simulink model "model"  (R2022b)
settings: Solver=VariableStepAuto  StartTime=0.0  StopTime=15  RelTol=1e-3
libraries: neural x114, simulink x4
(part 2 of 4)

== system model/level=2，训练时间15s，隐藏层15/Layer 1/Delays 1 ==
  "p{1}" : Inport  PortDimensions=8
      mask Display: e = 0.06;c1 = [120 230 180]/255;c2 = ([120 230 180]+0)/(256+128);c3 = ([120 230 180]+128)/(256+128);patch([0 1 1 0],[0 0 1 1],c1);patch([0 1 1 1-e 1-e 0+e],[0 0 1 1-e 0+e 0+e],c2);patch([0 0 1 1-e 0+e 0+e],[0 1 1 1-e 1-e 0+e],c3);plot([0 1 1 0 0],[0 0 1 1 0]);
  mux : Mux  Inputs=1
      mask Display: e = 0.06;c1 = [120 150 230]/255;c2 = ([120 150 230]+0)/383;c3 = ([120 150 230]+128)/383;patch([0 1 1 0],[0 0 1 1],c1);patch([0 1 1 1-e 1-e 0+e],[0 0 1 1-e 0+e 0+e],c2);patch([0 0 1 1-e 0+e 0+e],[0 1 1 1-e 1-e 0+e],c3);plot([0 1 1 0 0],[0 0 1 1 0]);disp('Mux')
  "pd{1,1}" : Outport
      mask Display: e = 0.06;c1 = [120 230 180]/255;c2 = ([120 230 180]+0)/(256+128);c3 = ([120 230 180]+128)/(256+128);patch([0 1 1 0],[0 0 1 1],c1);patch([0 1 1 1-e 1-e 0+e],[0 0 1 1-e 0+e 0+e],c2);patch([0 0 1 1-e 0+e 0+e],[0 1 1 1-e 1-e 0+e],c3);plot([0 1 1 0 0],[0 0 1 1 0]);
  wires:
  "p{1}"/1 -> mux/1
  mux/1 -> "pd{1,1}"/1

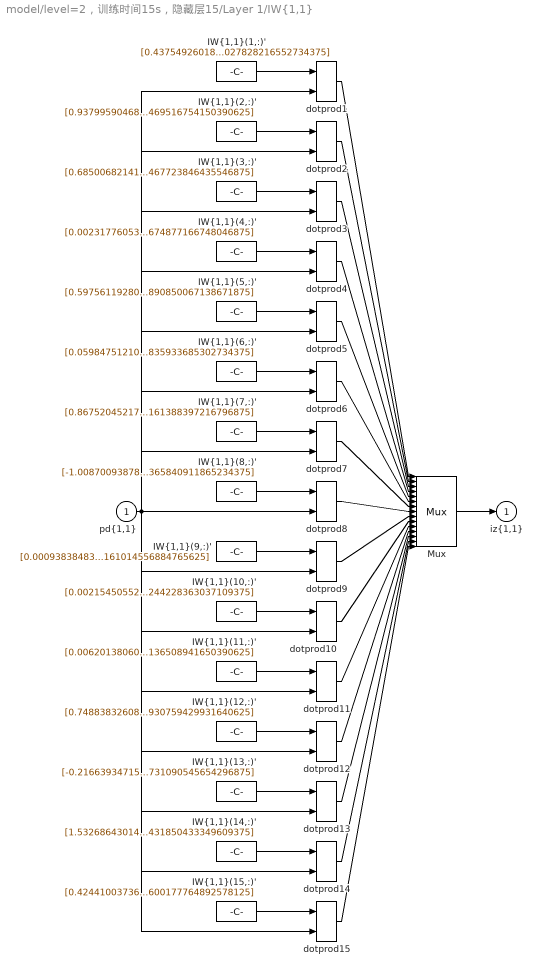
== system model/level=2，训练时间15s，隐藏层15/Layer 1/IW{1,1} ==
  "pd{1,1}" : Inport  PortDimensions=8
      mask Display: e = 0.06;c1 = [120 230 180]/255;c2 = ([120 230 180]+0)/(256+128);c3 = ([120 230 180]+128)/(256+128);patch([0 1 1 0],[0 0 1 1],c1);patch([0 1 1 1-e 1-e 0+e],[0 0 1 1-e 0+e 0+e],c2);patch([0 0 1 1-e 0+e 0+e],[0 1 1 1-e 1-e 0+e],c3);plot([0 1 1 0 0],[0 0 1 1 0]);
  "IW{1,1}(1,:)'" : Constant  Value=[0.437549260188033473095714498413144610822200775146484375;-0.543752134402809783608745419769547879695892333984375;-0.77263238466385486535870086299837566912174224853515625;0.7440170273308268633627449162304401397705078125;-1.41516521745081202965366173884831368923187255859375;1.2537441253925447615102939380449242889881134033203125;0.904308850719730106249016898800618946552276611328125;-0.56373674454161937230622925198986195027828216552734375]
      mask Display: e = 0.06;c1 = [120 150 230]/255;c2 = ([120 150 230]+0)/383;c3 = ([120 150 230]+128)/383;patch([0 1 1 0],[0 0 1 1],c1);patch([0 1 1 1-e 1-e 0+e],[0 0 1 1-e 0+e 0+e],c2);patch([0 0 1 1-e 0+e 0+e],[0 1 1 1-e 1-e 0+e],c3);plot([0 1 1 0 0],[0 0 1 1 0]);disp('Weights');
  "IW{1,1}(10,:)'" : Constant  Value=[0.0021545055257757681106689506833617997472174465656280517578125;-0.000689327560344079183322907322661876605707220733165740966796875;0.0025722441794928919099605391096474704681895673274993896484375;0.01018820606628951554173401206071503111161291599273681640625;0.250021595562128828849068895578966476023197174072265625;0.405128587531441264335541063701384700834751129150390625;-0.09831810982660001141386629797125351615250110626220703125;-0.498693163090770885670366396880126558244228363037109375]
      mask Display: e = 0.06;c1 = [120 150 230]/255;c2 = ([120 150 230]+0)/383;c3 = ([120 150 230]+128)/383;patch([0 1 1 0],[0 0 1 1],c1);patch([0 1 1 1-e 1-e 0+e],[0 0 1 1-e 0+e 0+e],c2);patch([0 0 1 1-e 0+e 0+e],[0 1 1 1-e 1-e 0+e],c3);plot([0 1 1 0 0],[0 0 1 1 0]);disp('Weights');
  "IW{1,1}(11,:)'" : Constant  Value=[0.006201380606661944898394533964847141760401427745819091796875;0.0037383409814706852584975660391819474170915782451629638671875;0.0040645559789425182717348405958546209149062633514404296875;0.0276355472342307249833393001381409703753888607025146484375;0.10749327599186429826882971383383846841752529144287109375;1.5640527442188096873820768450968898832798004150390625;0.364238376530578611411925749052898027002811431884765625;-1.772260716698662807999653523438610136508941650390625]
      mask Display: e = 0.06;c1 = [120 150 230]/255;c2 = ([120 150 230]+0)/383;c3 = ([120 150 230]+128)/383;patch([0 1 1 0],[0 0 1 1],c1);patch([0 1 1 1-e 1-e 0+e],[0 0 1 1-e 0+e 0+e],c2);patch([0 0 1 1-e 0+e 0+e],[0 1 1 1-e 1-e 0+e],c3);plot([0 1 1 0 0],[0 0 1 1 0]);disp('Weights');
  "IW{1,1}(12,:)'" : Constant  Value=[0.7488383260876163571850838707177899777889251708984375;1.484571579328911372641641719383187592029571533203125;0.16446117310405139466666923908633179962635040283203125;0.1800313451031676781344259552497533150017261505126953125;1.4197521021375887340099097855272702872753143310546875;0.5167645863546084239459332820842973887920379638671875;-0.83653735985908939110089477253495715558528900146484375;-0.4654659156868492519976143739768303930759429931640625]
      mask Display: e = 0.06;c1 = [120 150 230]/255;c2 = ([120 150 230]+0)/383;c3 = ([120 150 230]+128)/383;patch([0 1 1 0],[0 0 1 1],c1);patch([0 1 1 1-e 1-e 0+e],[0 0 1 1-e 0+e 0+e],c2);patch([0 0 1 1-e 0+e 0+e],[0 1 1 1-e 1-e 0+e],c3);plot([0 1 1 0 0],[0 0 1 1 0]);disp('Weights');
  "IW{1,1}(13,:)'" : Constant  Value=[-0.2166393471563960171355489592315279878675937652587890625;-0.72288634706720411582381302650901488959789276123046875;0.76398367116674703591883144326857291162014007568359375;0.31702488552167162882966522374772466719150543212890625;1.61289116019904898990944275283254683017730712890625;-0.6538957185094822488480303945834748446941375732421875;-1.731230912011282985218940666527487337589263916015625;-1.03061719525024653165701238322071731090545654296875]
      mask Display: e = 0.06;c1 = [120 150 230]/255;c2 = ([120 150 230]+0)/383;c3 = ([120 150 230]+128)/383;patch([0 1 1 0],[0 0 1 1],c1);patch([0 1 1 1-e 1-e 0+e],[0 0 1 1-e 0+e 0+e],c2);patch([0 0 1 1-e 0+e 0+e],[0 1 1 1-e 1-e 0+e],c3);plot([0 1 1 0 0],[0 0 1 1 0]);disp('Weights');
  "IW{1,1}(14,:)'" : Constant  Value=[1.532686430143353373267700590076856315135955810546875;1.384326577376502331873098228243179619312286376953125;-0.66610376092964418415220961833256296813488006591796875;-0.68326384700084352719073876869515515863895416259765625;2.42772285085268624271748194587416946887969970703125;-1.7746665444950675549762308946810662746429443359375;-3.146294986981688079907826249836944043636322021484375;4.184593075317817323366398341022431850433349609375]
      mask Display: e = 0.06;c1 = [120 150 230]/255;c2 = ([120 150 230]+0)/383;c3 = ([120 150 230]+128)/383;patch([0 1 1 0],[0 0 1 1],c1);patch([0 1 1 1-e 1-e 0+e],[0 0 1 1-e 0+e 0+e],c2);patch([0 0 1 1-e 0+e 0+e],[0 1 1 1-e 1-e 0+e],c3);plot([0 1 1 0 0],[0 0 1 1 0]);disp('Weights');
  "IW{1,1}(15,:)'" : Constant  Value=[0.42441003736812199509387255602632649242877960205078125;-0.317624639112158824172382765027577988803386688232421875;0.6566292418801129571193087031133472919464111328125;0.354371501508666864044272415412706322968006134033203125;0.55838469564761428198806925138342194259166717529296875;0.634921241532747426816740698995999991893768310546875;0.855102081342001607566771781421266496181488037109375;-2.10814001639689241329733704333193600177764892578125]
      mask Display: e = 0.06;c1 = [120 150 230]/255;c2 = ([120 150 230]+0)/383;c3 = ([120 150 230]+128)/383;patch([0 1 1 0],[0 0 1 1],c1);patch([0 1 1 1-e 1-e 0+e],[0 0 1 1-e 0+e 0+e],c2);patch([0 0 1 1-e 0+e 0+e],[0 1 1 1-e 1-e 0+e],c3);plot([0 1 1 0 0],[0 0 1 1 0]);disp('Weights');
  "IW{1,1}(2,:)'" : Constant  Value=[0.93799590468169125045960754505358636379241943359375;0.0389757109661090506147473888631793670356273651123046875;1.225492864464332143370484118349850177764892578125;-1.40774598885113988444572896696627140045166015625;-0.54987653716072848464335720564122311770915985107421875;-2.160972880697380471559654324664734303951263427734375;-0.1067846054083453621874610917075187899172306060791015625;0.4523584479950049086482977145351469516754150390625]
      mask Display: e = 0.06;c1 = [120 150 230]/255;c2 = ([120 150 230]+0)/383;c3 = ([120 150 230]+128)/383;patch([0 1 1 0],[0 0 1 1],c1);patch([0 1 1 1-e 1-e 0+e],[0 0 1 1-e 0+e 0+e],c2);patch([0 0 1 1-e 0+e 0+e],[0 1 1 1-e 1-e 0+e],c3);plot([0 1 1 0 0],[0 0 1 1 0]);disp('Weights');
  "IW{1,1}(3,:)'" : Constant  Value=[0.685006821417439848431740756495855748653411865234375;-0.151121840928223838407262746841297484934329986572265625;-0.90905729353138209347662268555723130702972412109375;-0.9146870439134369146216840817942284047603607177734375;1.5466948145383672130748209383455105125904083251953125;-1.0684967037827195479593456184375099837779998779296875;-1.41530069117394763367201449000276625156402587890625;2.208804266633716206769122436526231467723846435546875]
      mask Display: e = 0.06;c1 = [120 150 230]/255;c2 = ([120 150 230]+0)/383;c3 = ([120 150 230]+128)/383;patch([0 1 1 0],[0 0 1 1],c1);patch([0 1 1 1-e 1-e 0+e],[0 0 1 1-e 0+e 0+e],c2);patch([0 0 1 1-e 0+e 0+e],[0 1 1 1-e 1-e 0+e],c3);plot([0 1 1 0 0],[0 0 1 1 0]);disp('Weights');
  "IW{1,1}(4,:)'" : Constant  Value=[0.00231776053848237011123512019139525364153087139129638671875;-0.000436669150460885385246767587119620657176710665225982666015625;0.0025125418369684950244125065665912188705988228321075439453125;0.01191060627903158843088338159077466116286814212799072265625;0.53703993975591324261387171645765192806720733642578125;1.4164231725934055550197854245197959244251251220703125;-0.237965122046671695432706883366336114704608917236328125;-1.035250733950956014695066187414340674877166748046875]
      mask Display: e = 0.06;c1 = [120 150 230]/255;c2 = ([120 150 230]+0)/383;c3 = ([120 150 230]+128)/383;patch([0 1 1 0],[0 0 1 1],c1);patch([0 1 1 1-e 1-e 0+e],[0 0 1 1-e 0+e 0+e],c2);patch([0 0 1 1-e 0+e 0+e],[0 1 1 1-e 1-e 0+e],c3);plot([0 1 1 0 0],[0 0 1 1 0]);disp('Weights');
  "IW{1,1}(5,:)'" : Constant  Value=[0.59756119280919561820297758458764292299747467041015625;-0.6096022740572006881620836793445050716400146484375;-0.188502054741053637343384252744726836681365966796875;-0.08490586213242155844138636666684760712087154388427734375;-0.227815400909060550294071845200960524380207061767578125;0.347143384643888663898536606211564503610134124755859375;-1.9577073019096020711771188871352933347225189208984375;0.71978561343270797134863414612482301890850067138671875]
      mask Display: e = 0.06;c1 = [120 150 230]/255;c2 = ([120 150 230]+0)/383;c3 = ([120 150 230]+128)/383;patch([0 1 1 0],[0 0 1 1],c1);patch([0 1 1 1-e 1-e 0+e],[0 0 1 1-e 0+e 0+e],c2);patch([0 0 1 1-e 0+e 0+e],[0 1 1 1-e 1-e 0+e],c3);plot([0 1 1 0 0],[0 0 1 1 0]);disp('Weights');
  "IW{1,1}(6,:)'" : Constant  Value=[0.059847512100399909151793309547429089434444904327392578125;0.74983605040232192973093106047599576413631439208984375;-0.7210875241722394246579597165691666305065155029296875;1.047180192591222525066996240639127790927886962890625;0.07693879015290940037719025212936685420572757720947265625;1.741335040725929150795536770601756870746612548828125;0.07038197833113417345440865346972714178264141082763671875;0.09342308462036284788521101063452078960835933685302734375]
      mask Display: e = 0.06;c1 = [120 150 230]/255;c2 = ([120 150 230]+0)/383;c3 = ([120 150 230]+128)/383;patch([0 1 1 0],[0 0 1 1],c1);patch([0 1 1 1-e 1-e 0+e],[0 0 1 1-e 0+e 0+e],c2);patch([0 0 1 1-e 0+e 0+e],[0 1 1 1-e 1-e 0+e],c3);plot([0 1 1 0 0],[0 0 1 1 0]);disp('Weights');
  "IW{1,1}(7,:)'" : Constant  Value=[0.86752045217883433370076318169594742357730865478515625;-0.96548421997974731567637718399055302143096923828125;0.321899851156346006320063679595477879047393798828125;-1.0278579156471467914713002755888737738132476806640625;-0.1653280131719136736290209910293924622237682342529296875;1.3665634118383358508452829482848756015300750732421875;-0.653315092554610732378250759211368858814239501953125;-0.354784734114196698140375474395113997161388397216796875]
      mask Display: e = 0.06;c1 = [120 150 230]/255;c2 = ([120 150 230]+0)/383;c3 = ([120 150 230]+128)/383;patch([0 1 1 0],[0 0 1 1],c1);patch([0 1 1 1-e 1-e 0+e],[0 0 1 1-e 0+e 0+e],c2);patch([0 0 1 1-e 0+e 0+e],[0 1 1 1-e 1-e 0+e],c3);plot([0 1 1 0 0],[0 0 1 1 0]);disp('Weights');
  "IW{1,1}(8,:)'" : Constant  Value=[-1.0087009387896153089769768484984524548053741455078125;-0.89390992537081881419425144486012868583202362060546875;-1.1882265121192616685874554605106823146343231201171875;0.83809871162911953046403823464061133563518524169921875;-1.59123040137597282495107720023952424526214599609375;0.267739811475067812640560305226244963705539703369140625;2.231364372002818896589815267361700534820556640625;-0.58440227767868557773311977143748663365840911865234375]
      mask Display: e = 0.06;c1 = [120 150 230]/255;c2 = ([120 150 230]+0)/383;c3 = ([120 150 230]+128)/383;patch([0 1 1 0],[0 0 1 1],c1);patch([0 1 1 1-e 1-e 0+e],[0 0 1 1-e 0+e 0+e],c2);patch([0 0 1 1-e 0+e 0+e],[0 1 1 1-e 1-e 0+e],c3);plot([0 1 1 0 0],[0 0 1 1 0]);disp('Weights');
  "IW{1,1}(9,:)'" : Constant  Value=[0.000938384833547240893893148783178048688569106161594390869140625;-0.00012713226525252224632760167377654170195455662906169891357421875;0.000847236512902139614518415289268205015105195343494415283203125;0.005008163419334926529102869352527704904787242412567138671875;-0.65488636048362280916990130208432674407958984375;-0.158363103243627623140099558440851978957653045654296875;0.328358097555003503043025148144806735217571258544921875;-0.071767526744820619999387645293609239161014556884765625]
      mask Display: e = 0.06;c1 = [120 150 230]/255;c2 = ([120 150 230]+0)/383;c3 = ([120 150 230]+128)/383;patch([0 1 1 0],[0 0 1 1],c1);patch([0 1 1 1-e 1-e 0+e],[0 0 1 1-e 0+e 0+e],c2);patch([0 0 1 1-e 0+e 0+e],[0 1 1 1-e 1-e 0+e],c3);plot([0 1 1 0 0],[0 0 1 1 0]);disp('Weights');
  Mux : Mux  Inputs=15
      mask Display: e = 0.06;c1 = [120 150 230]/255;c2 = ([120 150 230]+0)/383;c3 = ([120 150 230]+128)/383;patch([0 1 1 0],[0 0 1 1],c1);patch([0 1 1 1-e 1-e 0+e],[0 0 1 1-e 0+e 0+e],c2);patch([0 0 1 1-e 0+e 0+e],[0 1 1 1-e 1-e 0+e],c3);plot([0 1 1 0 0],[0 0 1 1 0]);disp('Mux');
  dotprod{1..15} (15 alike) : neural/Weight Functions/dotprod
  "iz{1,1}" : Outport
      mask Display: e = 0.06;c1 = [120 230 180]/255;c2 = ([120 230 180]+0)/(256+128);c3 = ([120 230 180]+128)/(256+128);patch([0 1 1 0],[0 0 1 1],c1);patch([0 1 1 1-e 1-e 0+e],[0 0 1 1-e 0+e 0+e],c2);patch([0 0 1 1-e 0+e 0+e],[0 1 1 1-e 1-e 0+e],c3);plot([0 1 1 0 0],[0 0 1 1 0]);
  wires:
  "IW{1,1}(1,:)'"/1 -> dotprod1/1
  "pd{1,1}"/1 -> dotprod1/2, dotprod2/2, dotprod3/2, dotprod4/2, dotprod5/2, dotprod6/2, dotprod7/2, dotprod8/2, dotprod9/2, dotprod10/2, dotprod11/2, dotprod12/2, dotprod13/2, dotprod14/2, dotprod15/2
  dotprod1/1 -> Mux/1
  "IW{1,1}(2,:)'"/1 -> dotprod2/1
  dotprod2/1 -> Mux/2
  "IW{1,1}(3,:)'"/1 -> dotprod3/1
  dotprod3/1 -> Mux/3
  "IW{1,1}(4,:)'"/1 -> dotprod4/1
  dotprod4/1 -> Mux/4
  "IW{1,1}(5,:)'"/1 -> dotprod5/1
  dotprod5/1 -> Mux/5
  "IW{1,1}(6,:)'"/1 -> dotprod6/1
  dotprod6/1 -> Mux/6
  "IW{1,1}(7,:)'"/1 -> dotprod7/1
  dotprod7/1 -> Mux/7
  "IW{1,1}(8,:)'"/1 -> dotprod8/1
  dotprod8/1 -> Mux/8
  "IW{1,1}(9,:)'"/1 -> dotprod9/1
  dotprod9/1 -> Mux/9
  "IW{1,1}(10,:)'"/1 -> dotprod10/1
  dotprod10/1 -> Mux/10
  "IW{1,1}(11,:)'"/1 -> dotprod11/1
  dotprod11/1 -> Mux/11
  "IW{1,1}(12,:)'"/1 -> dotprod12/1
  dotprod12/1 -> Mux/12
  "IW{1,1}(13,:)'"/1 -> dotprod13/1
  dotprod13/1 -> Mux/13
  "IW{1,1}(14,:)'"/1 -> dotprod14/1
  dotprod14/1 -> Mux/14
  "IW{1,1}(15,:)'"/1 -> dotprod15/1
  dotprod15/1 -> Mux/15
  Mux/1 -> "iz{1,1}"/1

== system model/level=2，训练时间15s，隐藏层15/Layer 2/Delays 1 ==
  "p{2}" : Inport  PortDimensions=15
      mask Display: e = 0.06;c1 = [120 230 180]/255;c2 = ([120 230 180]+0)/(256+128);c3 = ([120 230 180]+128)/(256+128);patch([0 1 1 0],[0 0 1 1],c1);patch([0 1 1 1-e 1-e 0+e],[0 0 1 1-e 0+e 0+e],c2);patch([0 0 1 1-e 0+e 0+e],[0 1 1 1-e 1-e 0+e],c3);plot([0 1 1 0 0],[0 0 1 1 0]);
  mux : Mux  Inputs=1
      mask Display: e = 0.06;c1 = [120 150 230]/255;c2 = ([120 150 230]+0)/383;c3 = ([120 150 230]+128)/383;patch([0 1 1 0],[0 0 1 1],c1);patch([0 1 1 1-e 1-e 0+e],[0 0 1 1-e 0+e 0+e],c2);patch([0 0 1 1-e 0+e 0+e],[0 1 1 1-e 1-e 0+e],c3);plot([0 1 1 0 0],[0 0 1 1 0]);disp('Mux')
  "pd{2,1}" : Outport
      mask Display: e = 0.06;c1 = [120 230 180]/255;c2 = ([120 230 180]+0)/(256+128);c3 = ([120 230 180]+128)/(256+128);patch([0 1 1 0],[0 0 1 1],c1);patch([0 1 1 1-e 1-e 0+e],[0 0 1 1-e 0+e 0+e],c2);patch([0 0 1 1-e 0+e 0+e],[0 1 1 1-e 1-e 0+e],c3);plot([0 1 1 0 0],[0 0 1 1 0]);
  wires:
  "p{2}"/1 -> mux/1
  mux/1 -> "pd{2,1}"/1

== system model/level=2，训练时间15s，隐藏层15/Layer 2/LW{2,1} ==
  "ad{2,1}" : Inport  PortDimensions=15
      mask Display: e = 0.06;c1 = [120 230 180]/255;c2 = ([120 230 180]+0)/(256+128);c3 = ([120 230 180]+128)/(256+128);patch([0 1 1 0],[0 0 1 1],c1);patch([0 1 1 1-e 1-e 0+e],[0 0 1 1-e 0+e 0+e],c2);patch([0 0 1 1-e 0+e 0+e],[0 1 1 1-e 1-e 0+e],c3);plot([0 1 1 0 0],[0 0 1 1 0]);
  "IW{2,1}(1,:)'" : Constant  Value=[0.000348521019966015134679271358919550038990564644336700439453125;-0.00105511526222962464909016500058669407735578715801239013671875;-0.0004875548366492649652627344725175362327718175947666168212890625;-1.1162096356705231148254142681253142654895782470703125;0.000566277605183764984851657597886287476285360753536224365234375;0.000434593678046664758617134705076523459865711629390716552734375;-0.0003371799056245722465974257175957973231561481952667236328125;0.00021859886636651514632383175307239753237809054553508758544921875;-2.87625249739135568916026386432349681854248046875;2.514252278515631378041916832444258034229278564453125;0.346485318185967783310985623757005669176578521728515625;0.000561811409637976810586834641725317851523868739604949951171875;0.00014173139297834577601635508425914622421259991824626922607421875;-0.00010903110141313854101509372984679657747619785368442535400390625;-0.001096015330055519036711597635758153046481311321258544921875]
      mask Display: e = 0.06;c1 = [120 150 230]/255;c2 = ([120 150 230]+0)/383;c3 = ([120 150 230]+128)/383;patch([0 1 1 0],[0 0 1 1],c1);patch([0 1 1 1-e 1-e 0+e],[0 0 1 1-e 0+e 0+e],c2);patch([0 0 1 1-e 0+e 0+e],[0 1 1 1-e 1-e 0+e],c3);plot([0 1 1 0 0],[0 0 1 1 0]);disp('weights');
  "IW{2,1}(2,:)'" : Constant  Value=[-0.000118459432783138453857720018280730300830327905714511871337890625;0.00109455608219046775751726041647771126008592545986175537109375;0.000248773173976225663028838397394792991690337657928466796875;2.376139494105127258904985865228809416294097900390625;-0.00060637236490409629312281492019565121154300868511199951171875;-0.000489683042123572405575349097972548406687565147876739501953125;0.00023224171170072960106167681004762926022522151470184326171875;-0.0002224587961179582090535944427500680831144563853740692138671875;0.76265316778717873180681863232166506350040435791015625;-2.917666926702186191988630525884218513965606689453125;-0.389603751198402570299350600180332548916339874267578125;-0.000526230007708676397575053851340953769977204501628875732421875;-0.000272639471284036728586375186722534635919146239757537841796875;0.0001435751291894367159991674487429236251045949757099151611328125;0.001218926641691715773152537849455256946384906768798828125]
      mask Display: e = 0.06;c1 = [120 150 230]/255;c2 = ([120 150 230]+0)/383;c3 = ([120 150 230]+128)/383;patch([0 1 1 0],[0 0 1 1],c1);patch([0 1 1 1-e 1-e 0+e],[0 0 1 1-e 0+e 0+e],c2);patch([0 0 1 1-e 0+e 0+e],[0 1 1 1-e 1-e 0+e],c3);plot([0 1 1 0 0],[0 0 1 1 0]);disp('weights');
  Mux : Mux  Inputs=2
      mask Display: e = 0.06;c1 = [120 150 230]/255;c2 = ([120 150 230]+0)/383;c3 = ([120 150 230]+128)/383;patch([0 1 1 0],[0 0 1 1],c1);patch([0 1 1 1-e 1-e 0+e],[0 0 1 1-e 0+e 0+e],c2);patch([0 0 1 1-e 0+e 0+e],[0 1 1 1-e 1-e 0+e],c3);plot([0 1 1 0 0],[0 0 1 1 0]);disp('Mux');
  dotprod1 : neural/Weight Functions/dotprod
  dotprod2 : neural/Weight Functions/dotprod
  "lz{2,1}" : Outport
      mask Display: e = 0.06;c1 = [120 230 180]/255;c2 = ([120 230 180]+0)/(256+128);c3 = ([120 230 180]+128)/(256+128);patch([0 1 1 0],[0 0 1 1],c1);patch([0 1 1 1-e 1-e 0+e],[0 0 1 1-e 0+e 0+e],c2);patch([0 0 1 1-e 0+e 0+e],[0 1 1 1-e 1-e 0+e],c3);plot([0 1 1 0 0],[0 0 1 1 0]);
  wires:
  "IW{2,1}(1,:)'"/1 -> dotprod1/1
  "ad{2,1}"/1 -> dotprod1/2, dotprod2/2
  dotprod1/1 -> Mux/1
  "IW{2,1}(2,:)'"/1 -> dotprod2/1
  dotprod2/1 -> Mux/2
  Mux/1 -> "lz{2,1}"/1

== system model/level=2，训练时间15s，隐藏层30/Layer 1/Delays 1 ==
  "p{1}" : Inport  PortDimensions=8
      mask Display: e = 0.06;c1 = [120 230 180]/255;c2 = ([120 230 180]+0)/(256+128);c3 = ([120 230 180]+128)/(256+128);patch([0 1 1 0],[0 0 1 1],c1);patch([0 1 1 1-e 1-e 0+e],[0 0 1 1-e 0+e 0+e],c2);patch([0 0 1 1-e 0+e 0+e],[0 1 1 1-e 1-e 0+e],c3);plot([0 1 1 0 0],[0 0 1 1 0]);
  mux : Mux  Inputs=1
      mask Display: e = 0.06;c1 = [120 150 230]/255;c2 = ([120 150 230]+0)/383;c3 = ([120 150 230]+128)/383;patch([0 1 1 0],[0 0 1 1],c1);patch([0 1 1 1-e 1-e 0+e],[0 0 1 1-e 0+e 0+e],c2);patch([0 0 1 1-e 0+e 0+e],[0 1 1 1-e 1-e 0+e],c3);plot([0 1 1 0 0],[0 0 1 1 0]);disp('Mux')
  "pd{1,1}" : Outport
      mask Display: e = 0.06;c1 = [120 230 180]/255;c2 = ([120 230 180]+0)/(256+128);c3 = ([120 230 180]+128)/(256+128);patch([0 1 1 0],[0 0 1 1],c1);patch([0 1 1 1-e 1-e 0+e],[0 0 1 1-e 0+e 0+e],c2);patch([0 0 1 1-e 0+e 0+e],[0 1 1 1-e 1-e 0+e],c3);plot([0 1 1 0 0],[0 0 1 1 0]);
  wires:
  "p{1}"/1 -> mux/1
  mux/1 -> "pd{1,1}"/1

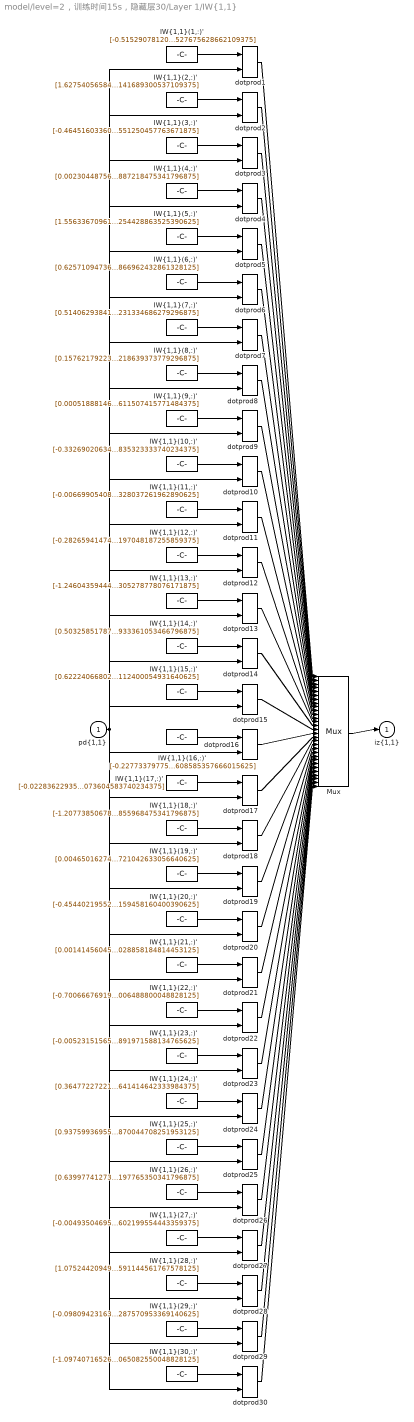
== system model/level=2，训练时间15s，隐藏层30/Layer 1/IW{1,1} ==
  "pd{1,1}" : Inport  PortDimensions=8
      mask Display: e = 0.06;c1 = [120 230 180]/255;c2 = ([120 230 180]+0)/(256+128);c3 = ([120 230 180]+128)/(256+128);patch([0 1 1 0],[0 0 1 1],c1);patch([0 1 1 1-e 1-e 0+e],[0 0 1 1-e 0+e 0+e],c2);patch([0 0 1 1-e 0+e 0+e],[0 1 1 1-e 1-e 0+e],c3);plot([0 1 1 0 0],[0 0 1 1 0]);
  "IW{1,1}(1,:)'" : Constant  Value=[-0.51529078120398874585106341328355483710765838623046875;-0.358908036286977927264985055444412864744663238525390625;-0.6444010451648869430840704808360897004604339599609375;1.0071702189204874144934365176595747470855712890625;0.02248108230128505191647292349443887360394001007080078125;0.26389261957038900874294995446689426898956298828125;-1.39021552883888066531881122500635683536529541015625;1.2659727968487819449450171305215917527675628662109375]
      mask Display: e = 0.06;c1 = [120 150 230]/255;c2 = ([120 150 230]+0)/383;c3 = ([120 150 230]+128)/383;patch([0 1 1 0],[0 0 1 1],c1);patch([0 1 1 1-e 1-e 0+e],[0 0 1 1-e 0+e 0+e],c2);patch([0 0 1 1-e 0+e 0+e],[0 1 1 1-e 1-e 0+e],c3);plot([0 1 1 0 0],[0 0 1 1 0]);disp('Weights');
  "IW{1,1}(10,:)'" : Constant  Value=[-0.332690206349311623501563417448778636753559112548828125;-0.446190121055760169355153266224078834056854248046875;-0.66273204507507565974577801171108148992061614990234375;0.28187276867938881874664502902305684983730316162109375;-0.189171155935518309210152665400528348982334136962890625;1.6197350687076081943160943410475738346576690673828125;0.56871889947271869747424943852820433676242828369140625;-0.255758907890911879601247846949263475835323333740234375]
      mask Display: e = 0.06;c1 = [120 150 230]/255;c2 = ([120 150 230]+0)/383;c3 = ([120 150 230]+128)/383;patch([0 1 1 0],[0 0 1 1],c1);patch([0 1 1 1-e 1-e 0+e],[0 0 1 1-e 0+e 0+e],c2);patch([0 0 1 1-e 0+e 0+e],[0 1 1 1-e 1-e 0+e],c3);plot([0 1 1 0 0],[0 0 1 1 0]);disp('Weights');
  "IW{1,1}(11,:)'" : Constant  Value=[-0.00669905408885207616365153882043159683234989643096923828125;7.324578259464768997637207359474587065051309764385223388671875e-05;0.005122104765875284786147414450852011214010417461395263671875;0.0044576255094989185312481794198902207426726818084716796875;-0.61000919335633485562908617794164456427097320556640625;0.87083644538918825173112736592884175479412078857421875;1.41342271393398188905621282174251973628997802734375;0.2003239174094197105890913235271000303328037261962890625]
      mask Display: e = 0.06;c1 = [120 150 230]/255;c2 = ([120 150 230]+0)/383;c3 = ([120 150 230]+128)/383;patch([0 1 1 0],[0 0 1 1],c1);patch([0 1 1 1-e 1-e 0+e],[0 0 1 1-e 0+e 0+e],c2);patch([0 0 1 1-e 0+e 0+e],[0 1 1 1-e 1-e 0+e],c3);plot([0 1 1 0 0],[0 0 1 1 0]);disp('Weights');
  "IW{1,1}(12,:)'" : Constant  Value=[-0.282659414743081705001515047115390188992023468017578125;-0.0262903330688668800119156543360077193938195705413818359375;-0.1239076488234570894153563358486280776560306549072265625;1.21520544753379855507091633626259863376617431640625;0.703174536692124707570883401785977184772491455078125;0.640376888760982865278492681682109832763671875;0.42448921427386909765999689625459723174571990966796875;-0.02889564638400710094856549403630197048187255859375]
      mask Display: e = 0.06;c1 = [120 150 230]/255;c2 = ([120 150 230]+0)/383;c3 = ([120 150 230]+128)/383;patch([0 1 1 0],[0 0 1 1],c1);patch([0 1 1 1-e 1-e 0+e],[0 0 1 1-e 0+e 0+e],c2);patch([0 0 1 1-e 0+e 0+e],[0 1 1 1-e 1-e 0+e],c3);plot([0 1 1 0 0],[0 0 1 1 0]);disp('Weights');
  "IW{1,1}(13,:)'" : Constant  Value=[-1.246043594448879243685723849921487271785736083984375;0.79398157078300923839009328730753622949123382568359375;-1.02458216852873551516722727683372795581817626953125;-0.16469520201554488370021545051713474094867706298828125;0.81489123823356701681319691488170064985752105712890625;0.9886847587319078645151648743194527924060821533203125;-1.3453903888704521474295461302972398698329925537109375;0.53475340518652003662936067485134117305278778076171875]
      mask Display: e = 0.06;c1 = [120 150 230]/255;c2 = ([120 150 230]+0)/383;c3 = ([120 150 230]+128)/383;patch([0 1 1 0],[0 0 1 1],c1);patch([0 1 1 1-e 1-e 0+e],[0 0 1 1-e 0+e 0+e],c2);patch([0 0 1 1-e 0+e 0+e],[0 1 1 1-e 1-e 0+e],c3);plot([0 1 1 0 0],[0 0 1 1 0]);disp('Weights');
  "IW{1,1}(14,:)'" : Constant  Value=[0.50325851787219788580074464334757067263126373291015625;1.274005584053836681590610169223509728908538818359375;0.1542261287740250008670983561387402005493640899658203125;-0.66552405816708015695581934778601862490177154541015625;0.11153763735982609450747560231320676393806934356689453125;-1.22764307291851171299867928610183298587799072265625;1.20325230730118004629503047908656299114227294921875;0.60351869658145307351304609255748800933361053466796875]
      mask Display: e = 0.06;c1 = [120 150 230]/255;c2 = ([120 150 230]+0)/383;c3 = ([120 150 230]+128)/383;patch([0 1 1 0],[0 0 1 1],c1);patch([0 1 1 1-e 1-e 0+e],[0 0 1 1-e 0+e 0+e],c2);patch([0 0 1 1-e 0+e 0+e],[0 1 1 1-e 1-e 0+e],c3);plot([0 1 1 0 0],[0 0 1 1 0]);disp('Weights');
  "IW{1,1}(15,:)'" : Constant  Value=[0.6222406680256307165421958416118286550045013427734375;0.25665149988952784543272400696878321468830108642578125;-0.7212900053632373964518365028197877109050750732421875;-1.0919638452088988866961472012917511165142059326171875;1.1517289607985954358326807778212241828441619873046875;0.47908070755476572788467137797852046787738800048828125;0.08229515016567899576838129860334447585046291351318359375;0.378045954995793354047606271706172265112400054931640625]
      mask Display: e = 0.06;c1 = [120 150 230]/255;c2 = ([120 150 230]+0)/383;c3 = ([120 150 230]+128)/383;patch([0 1 1 0],[0 0 1 1],c1);patch([0 1 1 1-e 1-e 0+e],[0 0 1 1-e 0+e 0+e],c2);patch([0 0 1 1-e 0+e 0+e],[0 1 1 1-e 1-e 0+e],c3);plot([0 1 1 0 0],[0 0 1 1 0]);disp('Weights');
  "IW{1,1}(16,:)'" : Constant  Value=[-0.2277337977585942863090195942277205176651477813720703125;-1.2779199309232840420236243517138063907623291015625;-0.65714457368775291978835184636409394443035125732421875;-1.0956903133672117878205654051271267235279083251953125;-0.75586952894212744435975537271588109433650970458984375;-0.32907615436963444377482801428413949906826019287109375;0.0159797887269795164943975152027633157558739185333251953125;0.43142324552849997676418070113868452608585357666015625]
      mask Display: e = 0.06;c1 = [120 150 230]/255;c2 = ([120 150 230]+0)/383;c3 = ([120 150 230]+128)/383;patch([0 1 1 0],[0 0 1 1],c1);patch([0 1 1 1-e 1-e 0+e],[0 0 1 1-e 0+e 0+e],c2);patch([0 0 1 1-e 0+e 0+e],[0 1 1 1-e 1-e 0+e],c3);plot([0 1 1 0 0],[0 0 1 1 0]);disp('Weights');
  "IW{1,1}(17,:)'" : Constant  Value=[-0.022836229354074942532459857602589181624352931976318359375;0.004580337135601772295678824065134904230944812297821044921875;-0.140173679995778843743181596437352709472179412841796875;-0.0854308094419960750709464036845020018517971038818359375;-0.4962848570689109006792705258703790605068206787109375;1.1265236830667435530273223776021040976047515869140625;-0.334325280814860736899873927541193552315235137939453125;0.1273758048059026870557630672919913195073604583740234375]
      mask Display: e = 0.06;c1 = [120 150 230]/255;c2 = ([120 150 230]+0)/383;c3 = ([120 150 230]+128)/383;patch([0 1 1 0],[0 0 1 1],c1);patch([0 1 1 1-e 1-e 0+e],[0 0 1 1-e 0+e 0+e],c2);patch([0 0 1 1-e 0+e 0+e],[0 1 1 1-e 1-e 0+e],c3);plot([0 1 1 0 0],[0 0 1 1 0]);disp('Weights');
  "IW{1,1}(18,:)'" : Constant  Value=[-1.2077385067840593624310940867871977388858795166015625;1.1674889928304581498963443664251826703548431396484375;0.09010823425861998192676338703677174635231494903564453125;0.449309159029992744027737217038520611822605133056640625;-0.57184806896710405066386329053784720599651336669921875;-0.1743456328312171510486194847544538788497447967529296875;-0.2325462740509626480278626559083932079374790191650390625;0.53695475722544461216756417343276552855968475341796875]
      mask Display: e = 0.06;c1 = [120 150 230]/255;c2 = ([120 150 230]+0)/383;c3 = ([120 150 230]+128)/383;patch([0 1 1 0],[0 0 1 1],c1);patch([0 1 1 1-e 1-e 0+e],[0 0 1 1-e 0+e 0+e],c2);patch([0 0 1 1-e 0+e 0+e],[0 1 1 1-e 1-e 0+e],c3);plot([0 1 1 0 0],[0 0 1 1 0]);disp('Weights');
  "IW{1,1}(19,:)'" : Constant  Value=[0.004650162746120789503123660324490629136562347412109375;0.0234561547946017974475285683411129866726696491241455078125;-0.438416575112286377446935148327611386775970458984375;-0.1686218033481821920727128372163861058652400970458984375;-0.58167516856673273650812916457653045654296875;0.82809358826238643747075229839538224041461944580078125;-1.184063328006768056610553685459308326244354248046875;1.27567234000135787397312014945782721042633056640625]
      mask Display: e = 0.06;c1 = [120 150 230]/255;c2 = ([120 150 230]+0)/383;c3 = ([120 150 230]+128)/383;patch([0 1 1 0],[0 0 1 1],c1);patch([0 1 1 1-e 1-e 0+e],[0 0 1 1-e 0+e 0+e],c2);patch([0 0 1 1-e 0+e 0+e],[0 1 1 1-e 1-e 0+e],c3);plot([0 1 1 0 0],[0 0 1 1 0]);disp('Weights');
  "IW{1,1}(2,:)'" : Constant  Value=[1.6275405658499126904104059576638974249362945556640625;-0.400817830235323857568374705806490965187549591064453125;-0.1498042860745256443788520073212566785514354705810546875;0.5680848416977768433611117870896123349666595458984375;-0.66152355799433315564073154746438376605510711669921875;-0.900875503135039945590278875897638499736785888671875;-0.1827509540485765804351814267647569067776203155517578125;-0.2033702569576057717082306908196187578141689300537109375]
      mask Display: e = 0.06;c1 = [120 150 230]/255;c2 = ([120 150 230]+0)/383;c3 = ([120 150 230]+128)/383;patch([0 1 1 0],[0 0 1 1],c1);patch([0 1 1 1-e 1-e 0+e],[0 0 1 1-e 0+e 0+e],c2);patch([0 0 1 1-e 0+e 0+e],[0 1 1 1-e 1-e 0+e],c3);plot([0 1 1 0 0],[0 0 1 1 0]);disp('Weights');
  "IW{1,1}(20,:)'" : Constant  Value=[-0.454402195521560747781819600277231074869632720947265625;0.757200677923064890961768469423986971378326416015625;-1.027225313862516475893471579183824360370635986328125;-1.5078137503128827834331104895682074129581451416015625;0.89172821423451364974965827059349976480007171630859375;-0.0214589518084518406093597064909772598184645175933837890625;-0.2767806396153476011789962285547517240047454833984375;0.649300414929707248035128941410221159458160400390625]
      mask Display: e = 0.06;c1 = [120 150 230]/255;c2 = ([120 150 230]+0)/383;c3 = ([120 150 230]+128)/383;patch([0 1 1 0],[0 0 1 1],c1);patch([0 1 1 1-e 1-e 0+e],[0 0 1 1-e 0+e 0+e],c2);patch([0 0 1 1-e 0+e 0+e],[0 1 1 1-e 1-e 0+e],c3);plot([0 1 1 0 0],[0 0 1 1 0]);disp('Weights');
  "IW{1,1}(21,:)'" : Constant  Value=[0.00141456045845024937050726787646226512151770293712615966796875;0.0020537989622576697211486784766520941047929227352142333984375;0.015745862357257937869103869843456777743995189666748046875;0.01163255540745552867043510758549018646590411663055419921875;-0.05628959906526591339126497359757195226848125457763671875;0.5106305317414492339622711369884200394153594970703125;0.42281814237427195468654872456681914627552032470703125;0.32290486466919265939878869176027365028858184814453125]
      mask Display: e = 0.06;c1 = [120 150 230]/255;c2 = ([120 150 230]+0)/383;c3 = ([120 150 230]+128)/383;patch([0 1 1 0],[0 0 1 1],c1);patch([0 1 1 1-e 1-e 0+e],[0 0 1 1-e 0+e 0+e],c2);patch([0 0 1 1-e 0+e 0+e],[0 1 1 1-e 1-e 0+e],c3);plot([0 1 1 0 0],[0 0 1 1 0]);disp('Weights');
  "IW{1,1}(22,:)'" : Constant  Value=[-0.70066676919565351600027724998653866350650787353515625;-0.08516496334898503162147420653127483092248439788818359375;1.070836165251404903386855949065648019313812255859375;-0.62143201396608294118095727753825485706329345703125;0.2667540680025772825700869361753575503826141357421875;1.1038269294929061725696328721824102103710174560546875;0.32438650498982568581851637645740993320941925048828125;0.835160372347516943847267611999996006488800048828125]
      mask Display: e = 0.06;c1 = [120 150 230]/255;c2 = ([120 150 230]+0)/383;c3 = ([120 150 230]+128)/383;patch([0 1 1 0],[0 0 1 1],c1);patch([0 1 1 1-e 1-e 0+e],[0 0 1 1-e 0+e 0+e],c2);patch([0 0 1 1-e 0+e 0+e],[0 1 1 1-e 1-e 0+e],c3);plot([0 1 1 0 0],[0 0 1 1 0]);disp('Weights');
  "IW{1,1}(23,:)'" : Constant  Value=[-0.005231515650782707187171904905653718742541968822479248046875;0.00120570690076083632778780607708313254988752305507659912109375;0.0139551835606677478163195615934455418027937412261962890625;0.01026685125497163453278659517309279181063175201416015625;1.0864845715929429825763463668408803641796112060546875;1.671183862644841422451236212509684264659881591796875;0.69484937898442733494874801181140355765819549560546875;0.137652130597095467834378723637200891971588134765625]
      mask Display: e = 0.06;c1 = [120 150 230]/255;c2 = ([120 150 230]+0)/383;c3 = ([120 150 230]+128)/383;patch([0 1 1 0],[0 0 1 1],c1);patch([0 1 1 1-e 1-e 0+e],[0 0 1 1-e 0+e 0+e],c2);patch([0 0 1 1-e 0+e 0+e],[0 1 1 1-e 1-e 0+e],c3);plot([0 1 1 0 0],[0 0 1 1 0]);disp('Weights');
  "IW{1,1}(24,:)'" : Constant  Value=[0.36477227221462193984535815616254694759845733642578125;-0.89430995801205270812062053664703853428363800048828125;-0.74976007337597450064237136757583357393741607666015625;1.1567893489832723474819431430660188198089599609375;-0.31622089930533492374564730198471806943416595458984375;0.65231064613815836761290256617940030992031097412109375;-0.0280945906075962988091010430480309878475964069366455078125;-0.278436234087035161532952542984276078641414642333984375]
      mask Display: e = 0.06;c1 = [120 150 230]/255;c2 = ([120 150 230]+0)/383;c3 = ([120 150 230]+128)/383;patch([0 1 1 0],[0 0 1 1],c1);patch([0 1 1 1-e 1-e 0+e],[0 0 1 1-e 0+e 0+e],c2);patch([0 0 1 1-e 0+e 0+e],[0 1 1 1-e 1-e 0+e],c3);plot([0 1 1 0 0],[0 0 1 1 0]);disp('Weights');
  "IW{1,1}(25,:)'" : Constant  Value=[0.93759936955434597383174377682735212147235870361328125;-0.491154337841410659759588952510966919362545013427734375;1.0978661121318340487817977191298268735408782958984375;0.046974507514647594053069923347720759920775890350341796875;0.96650258402587685413465123929199762642383575439453125;-0.47054605623098044731023037456907331943511962890625;-0.2164328978741686670961286154124536551535129547119140625;0.55316632141533805810951207604375667870044708251953125]
      mask Display: e = 0.06;c1 = [120 150 230]/255;c2 = ([120 150 230]+0)/383;c3 = ([120 150 230]+128)/383;patch([0 1 1 0],[0 0 1 1],c1);patch([0 1 1 1-e 1-e 0+e],[0 0 1 1-e 0+e 0+e],c2);patch([0 0 1 1-e 0+e 0+e],[0 1 1 1-e 1-e 0+e],c3);plot([0 1 1 0 0],[0 0 1 1 0]);disp('Weights');
  "IW{1,1}(26,:)'" : Constant  Value=[0.6399774127301880444207426990033127367496490478515625;-0.336440329936761040041659498456283472478389739990234375;-0.2282562353792261522489326353024807758629322052001953125;0.73086019314017403036842779329163022339344024658203125;-0.10640176537687706659340847181738354265689849853515625;0.05780691020579768746312510074858437292277812957763671875;-1.2687555849784306616356843733228743076324462890625;0.886819602665400719132549056666903197765350341796875]
      mask Display: e = 0.06;c1 = [120 150 230]/255;c2 = ([120 150 230]+0)/383;c3 = ([120 150 230]+128)/383;patch([0 1 1 0],[0 0 1 1],c1);patch([0 1 1 1-e 1-e 0+e],[0 0 1 1-e 0+e 0+e],c2);patch([0 0 1 1-e 0+e 0+e],[0 1 1 1-e 1-e 0+e],c3);plot([0 1 1 0 0],[0 0 1 1 0]);disp('Weights');
  "IW{1,1}(27,:)'" : Constant  Value=[-0.0049350469570973824751103364860682631842792034149169921875;0.000872830306299430375670256321285478406934998929500579833984375;0.0136548777400290095862533945592076634056866168975830078125;0.009413680004674830625877035572557360865175724029541015625;-0.54354708947521945816561128594912588596343994140625;1.05611502607035845358041115105152130126953125;1.3501917836071533063346805647597648203372955322265625;0.5384615968772690219878995776525698602199554443359375]
      mask Display: e = 0.06;c1 = [120 150 230]/255;c2 = ([120 150 230]+0)/383;c3 = ([120 150 230]+128)/383;patch([0 1 1 0],[0 0 1 1],c1);patch([0 1 1 1-e 1-e 0+e],[0 0 1 1-e 0+e 0+e],c2);patch([0 0 1 1-e 0+e 0+e],[0 1 1 1-e 1-e 0+e],c3);plot([0 1 1 0 0],[0 0 1 1 0]);disp('Weights');
  "IW{1,1}(28,:)'" : Constant  Value=[1.0752442094901144553631411326932720839977264404296875;0.1432570132179038224773393039868096821010112762451171875;0.64864287152507060785211479014833457767963409423828125;1.10512462758548135610681129037402570247650146484375;1.1870661129729882521388617533375509083271026611328125;-0.67416973342293118331980394941638223826885223388671875;-0.63829960082498826690056148436269722878932952880859375;0.39063849673528416861501000312273390591144561767578125]
      mask Display: e = 0.06;c1 = [120 150 230]/255;c2 = ([120 150 230]+0)/383;c3 = ([120 150 230]+128)/383;patch([0 1 1 0],[0 0 1 1],c1);patch([0 1 1 1-e 1-e 0+e],[0 0 1 1-e 0+e 0+e],c2);patch([0 0 1 1-e 0+e 0+e],[0 1 1 1-e 1-e 0+e],c3);plot([0 1 1 0 0],[0 0 1 1 0]);disp('Weights');
  "IW{1,1}(29,:)'" : Constant  Value=[-0.0980942316396304636594294379392522387206554412841796875;0.61189153107853655466641384919057600200176239013671875;-0.84566504371533779416125753414235077798366546630859375;0.0927520921897242167641906007702345959842205047607421875;-0.26913358286188115986448110561468638479709625244140625;0.62806592889813306346269428104278631508350372314453125;-0.289556931591415211979523292029625736176967620849609375;0.91556062789163039639106500544585287570953369140625]
      mask Display: e = 0.06;c1 = [120 150 230]/255;c2 = ([120 150 230]+0)/383;c3 = ([120 150 230]+128)/383;patch([0 1 1 0],[0 0 1 1],c1);patch([0 1 1 1-e 1-e 0+e],[0 0 1 1-e 0+e 0+e],c2);patch([0 0 1 1-e 0+e 0+e],[0 1 1 1-e 1-e 0+e],c3);plot([0 1 1 0 0],[0 0 1 1 0]);disp('Weights');
  "IW{1,1}(3,:)'" : Constant  Value=[-0.4645160336037006398868243195465765893459320068359375;-0.318029631620533492775138029173831455409526824951171875;-0.243538342681982877824253819198929704725742340087890625;-0.18946760705949283742910438377293758094310760498046875;0.8850916714125964812609481668914668262004852294921875;-0.05046766029266565312116910035911132581532001495361328125;0.223173470635031734321529484077473171055316925048828125;-0.319286815472195950604827885399572551250457763671875]
      mask Display: e = 0.06;c1 = [120 150 230]/255;c2 = ([120 150 230]+0)/383;c3 = ([120 150 230]+128)/383;patch([0 1 1 0],[0 0 1 1],c1);patch([0 1 1 1-e 1-e 0+e],[0 0 1 1-e 0+e 0+e],c2);patch([0 0 1 1-e 0+e 0+e],[0 1 1 1-e 1-e 0+e],c3);plot([0 1 1 0 0],[0 0 1 1 0]);disp('Weights');
  "IW{1,1}(30,:)'" : Constant  Value=[-1.097407165269583373401474091224372386932373046875;-0.94384304183028644441577625912032090127468109130859375;-0.41982421564875471720057475977228023111820220947265625;-0.74197266553401430844161268396419472992420196533203125;-0.07316610980940684016982089588054805062711238861083984375;-0.76977283374588034714491868726327084004878997802734375;0.75780678510813348491836904941010288894176483154296875;-0.0387446338690096425683151437624474056065082550048828125]
      mask Display: e = 0.06;c1 = [120 150 230]/255;c2 = ([120 150 230]+0)/383;c3 = ([120 150 230]+128)/383;patch([0 1 1 0],[0 0 1 1],c1);patch([0 1 1 1-e 1-e 0+e],[0 0 1 1-e 0+e 0+e],c2);patch([0 0 1 1-e 0+e 0+e],[0 1 1 1-e 1-e 0+e],c3);plot([0 1 1 0 0],[0 0 1 1 0]);disp('Weights');
  "IW{1,1}(4,:)'" : Constant  Value=[0.0023044875616817649295609005122287271660752594470977783203125;0.0013031975620043279202875385891502446611411869525909423828125;0.01072978657909527851199715797747558099217712879180908203125;0.00730618236334330296843919683169588097371160984039306640625;0.02017858238960852645949017869497765786945819854736328125;-1.5017058798047282497378773769014514982700347900390625;0.07980369228943810788745594209103728644549846649169921875;1.042604050993350295328809806960634887218475341796875]
      mask Display: e = 0.06;c1 = [120 150 230]/255;c2 = ([120 150 230]+0)/383;c3 = ([120 150 230]+128)/383;patch([0 1 1 0],[0 0 1 1],c1);patch([0 1 1 1-e 1-e 0+e],[0 0 1 1-e 0+e 0+e],c2);patch([0 0 1 1-e 0+e 0+e],[0 1 1 1-e 1-e 0+e],c3);plot([0 1 1 0 0],[0 0 1 1 0]);disp('Weights');
  "IW{1,1}(5,:)'" : Constant  Value=[1.5563367096133380318434547007200308144092559814453125;-0.80637828023243363073646605698741041123867034912109375;1.6731471994056377194937113017658703029155731201171875;-0.476306787625900673877055169214145280420780181884765625;-0.51322902231079947643621608222019858658313751220703125;0.298930635217688311922046295876498334109783172607421875;0.0656532703580477161597883650756557472050189971923828125;-1.3903319079435301208746977863484062254428863525390625]
      mask Display: e = 0.06;c1 = [120 150 230]/255;c2 = ([120 150 230]+0)/383;c3 = ([120 150 230]+128)/383;patch([0 1 1 0],[0 0 1 1],c1);patch([0 1 1 1-e 1-e 0+e],[0 0 1 1-e 0+e 0+e],c2);patch([0 0 1 1-e 0+e 0+e],[0 1 1 1-e 1-e 0+e],c3);plot([0 1 1 0 0],[0 0 1 1 0]);disp('Weights');
  "IW{1,1}(6,:)'" : Constant  Value=[0.6257109473685227296613220460130833089351654052734375;0.76605646991223519393088281503878533840179443359375;1.0287586493195808312606231993413530290126800537109375;-0.5168146738757084523996354619157500565052032470703125;0.6241740486004072607784110005013644695281982421875;1.8272670852487582493495210655964910984039306640625;0.1611670528065480556545452373029547743499279022216796875;-0.76430121610802104203941098603536374866962432861328125]
      mask Display: e = 0.06;c1 = [120 150 230]/255;c2 = ([120 150 230]+0)/383;c3 = ([120 150 230]+128)/383;patch([0 1 1 0],[0 0 1 1],c1);patch([0 1 1 1-e 1-e 0+e],[0 0 1 1-e 0+e 0+e],c2);patch([0 0 1 1-e 0+e 0+e],[0 1 1 1-e 1-e 0+e],c3);plot([0 1 1 0 0],[0 0 1 1 0]);disp('Weights');
  "IW{1,1}(7,:)'" : Constant  Value=[0.51406293841673422750915278811589814722537994384765625;0.4847358120104321432819460824248380959033966064453125;-0.7433515460789827944410035343025811016559600830078125;-1.023336638768546524858038537786342203617095947265625;0.5423219865939976624957807871396653354167938232421875;0.1325813261552004906906887526929494924843311309814453125;0.75558177437272278087476706787128932774066925048828125;-1.1122049706192373985658150559174828231334686279296875]
      mask Display: e = 0.06;c1 = [120 150 230]/255;c2 = ([120 150 230]+0)/383;c3 = ([120 150 230]+128)/383;patch([0 1 1 0],[0 0 1 1],c1);patch([0 1 1 1-e 1-e 0+e],[0 0 1 1-e 0+e 0+e],c2);patch([0 0 1 1-e 0+e 0+e],[0 1 1 1-e 1-e 0+e],c3);plot([0 1 1 0 0],[0 0 1 1 0]);disp('Weights');
  "IW{1,1}(8,:)'" : Constant  Value=[0.1576217922398347182078026662566117011010646820068359375;0.2433195239129355702534240890599903650581836700439453125;0.59468236315515099477124749682843685150146484375;0.74484365669387508912535622584982775151729583740234375;0.95528370076268787070006283101974986493587493896484375;-0.049323971997740197192872102505134535022079944610595703125;-0.8991187823153279357057954257470555603504180908203125;-1.346741965091527770681523179518990218639373779296875]
      mask Display: e = 0.06;c1 = [120 150 230]/255;c2 = ([120 150 230]+0)/383;c3 = ([120 150 230]+128)/383;patch([0 1 1 0],[0 0 1 1],c1);patch([0 1 1 1-e 1-e 0+e],[0 0 1 1-e 0+e 0+e],c2);patch([0 0 1 1-e 0+e 0+e],[0 1 1 1-e 1-e 0+e],c3);plot([0 1 1 0 0],[0 0 1 1 0]);disp('Weights');
  "IW{1,1}(9,:)'" : Constant  Value=[0.0005188814642104054748739105917820779723115265369415283203125;0.000780494294782365792724487807419109230977483093738555908203125;0.003766091858539578896003519048463203944265842437744140625;0.00179481972526165695254463106067532862653024494647979736328125;-0.0669846049372191665316478292879764921963214874267578125;-1.26682866540850991299294037162326276302337646484375;0.1426391260016890150108537227424676530063152313232421875;0.806183734345397251530584981082938611507415771484375]
      mask Display: e = 0.06;c1 = [120 150 230]/255;c2 = ([120 150 230]+0)/383;c3 = ([120 150 230]+128)/383;patch([0 1 1 0],[0 0 1 1],c1);patch([0 1 1 1-e 1-e 0+e],[0 0 1 1-e 0+e 0+e],c2);patch([0 0 1 1-e 0+e 0+e],[0 1 1 1-e 1-e 0+e],c3);plot([0 1 1 0 0],[0 0 1 1 0]);disp('Weights');
  Mux : Mux  Inputs=30
      mask Display: e = 0.06;c1 = [120 150 230]/255;c2 = ([120 150 230]+0)/383;c3 = ([120 150 230]+128)/383;patch([0 1 1 0],[0 0 1 1],c1);patch([0 1 1 1-e 1-e 0+e],[0 0 1 1-e 0+e 0+e],c2);patch([0 0 1 1-e 0+e 0+e],[0 1 1 1-e 1-e 0+e],c3);plot([0 1 1 0 0],[0 0 1 1 0]);disp('Mux');
  dotprod{1..30} (30 alike) : neural/Weight Functions/dotprod
  "iz{1,1}" : Outport
      mask Display: e = 0.06;c1 = [120 230 180]/255;c2 = ([120 230 180]+0)/(256+128);c3 = ([120 230 180]+128)/(256+128);patch([0 1 1 0],[0 0 1 1],c1);patch([0 1 1 1-e 1-e 0+e],[0 0 1 1-e 0+e 0+e],c2);patch([0 0 1 1-e 0+e 0+e],[0 1 1 1-e 1-e 0+e],c3);plot([0 1 1 0 0],[0 0 1 1 0]);
  wires:
  "IW{1,1}(1,:)'"/1 -> dotprod1/1
  "pd{1,1}"/1 -> dotprod1/2, dotprod2/2, dotprod3/2, dotprod4/2, dotprod5/2, dotprod6/2, dotprod7/2, dotprod8/2, dotprod9/2, dotprod10/2, dotprod11/2, dotprod12/2, dotprod13/2, dotprod14/2, dotprod15/2, dotprod16/2, dotprod17/2, dotprod18/2, dotprod19/2, dotprod20/2, dotprod21/2, dotprod22/2, dotprod23/2, dotprod24/2, dotprod25/2, dotprod26/2, dotprod27/2, dotprod28/2, dotprod29/2, dotprod30/2
  dotprod1/1 -> Mux/1
  "IW{1,1}(2,:)'"/1 -> dotprod2/1
  dotprod2/1 -> Mux/2
  "IW{1,1}(3,:)'"/1 -> dotprod3/1
  dotprod3/1 -> Mux/3
  "IW{1,1}(4,:)'"/1 -> dotprod4/1
  dotprod4/1 -> Mux/4
  "IW{1,1}(5,:)'"/1 -> dotprod5/1
  dotprod5/1 -> Mux/5
  "IW{1,1}(6,:)'"/1 -> dotprod6/1
  dotprod6/1 -> Mux/6
  "IW{1,1}(7,:)'"/1 -> dotprod7/1
  dotprod7/1 -> Mux/7
  "IW{1,1}(8,:)'"/1 -> dotprod8/1
  dotprod8/1 -> Mux/8
  "IW{1,1}(9,:)'"/1 -> dotprod9/1
  dotprod9/1 -> Mux/9
  "IW{1,1}(10,:)'"/1 -> dotprod10/1
  dotprod10/1 -> Mux/10
  "IW{1,1}(11,:)'"/1 -> dotprod11/1
  dotprod11/1 -> Mux/11
  "IW{1,1}(12,:)'"/1 -> dotprod12/1
  dotprod12/1 -> Mux/12
  "IW{1,1}(13,:)'"/1 -> dotprod13/1
  dotprod13/1 -> Mux/13
  "IW{1,1}(14,:)'"/1 -> dotprod14/1
  dotprod14/1 -> Mux/14
  "IW{1,1}(15,:)'"/1 -> dotprod15/1
  dotprod15/1 -> Mux/15
  "IW{1,1}(16,:)'"/1 -> dotprod16/1
  dotprod16/1 -> Mux/16
  "IW{1,1}(17,:)'"/1 -> dotprod17/1
  dotprod17/1 -> Mux/17
  "IW{1,1}(18,:)'"/1 -> dotprod18/1
  dotprod18/1 -> Mux/18
  "IW{1,1}(19,:)'"/1 -> dotprod19/1
  dotprod19/1 -> Mux/19
  "IW{1,1}(20,:)'"/1 -> dotprod20/1
  dotprod20/1 -> Mux/20
  "IW{1,1}(21,:)'"/1 -> dotprod21/1
  dotprod21/1 -> Mux/21
  "IW{1,1}(22,:)'"/1 -> dotprod22/1
  dotprod22/1 -> Mux/22
  "IW{1,1}(23,:)'"/1 -> dotprod23/1
  dotprod23/1 -> Mux/23
  "IW{1,1}(24,:)'"/1 -> dotprod24/1
  dotprod24/1 -> Mux/24
  "IW{1,1}(25,:)'"/1 -> dotprod25/1
  dotprod25/1 -> Mux/25
  "IW{1,1}(26,:)'"/1 -> dotprod26/1
  dotprod26/1 -> Mux/26
  "IW{1,1}(27,:)'"/1 -> dotprod27/1
  dotprod27/1 -> Mux/27
  "IW{1,1}(28,:)'"/1 -> dotprod28/1
  dotprod28/1 -> Mux/28
  "IW{1,1}(29,:)'"/1 -> dotprod29/1
  dotprod29/1 -> Mux/29
  "IW{1,1}(30,:)'"/1 -> dotprod30/1
  dotprod30/1 -> Mux/30
  Mux/1 -> "iz{1,1}"/1

== system model/level=2，训练时间15s，隐藏层30/Layer 2/Delays 1 ==
  "p{2}" : Inport  PortDimensions=30
      mask Display: e = 0.06;c1 = [120 230 180]/255;c2 = ([120 230 180]+0)/(256+128);c3 = ([120 230 180]+128)/(256+128);patch([0 1 1 0],[0 0 1 1],c1);patch([0 1 1 1-e 1-e 0+e],[0 0 1 1-e 0+e 0+e],c2);patch([0 0 1 1-e 0+e 0+e],[0 1 1 1-e 1-e 0+e],c3);plot([0 1 1 0 0],[0 0 1 1 0]);
  mux : Mux  Inputs=1
      mask Display: e = 0.06;c1 = [120 150 230]/255;c2 = ([120 150 230]+0)/383;c3 = ([120 150 230]+128)/383;patch([0 1 1 0],[0 0 1 1],c1);patch([0 1 1 1-e 1-e 0+e],[0 0 1 1-e 0+e 0+e],c2);patch([0 0 1 1-e 0+e 0+e],[0 1 1 1-e 1-e 0+e],c3);plot([0 1 1 0 0],[0 0 1 1 0]);disp('Mux')
  "pd{2,1}" : Outport
      mask Display: e = 0.06;c1 = [120 230 180]/255;c2 = ([120 230 180]+0)/(256+128);c3 = ([120 230 180]+128)/(256+128);patch([0 1 1 0],[0 0 1 1],c1);patch([0 1 1 1-e 1-e 0+e],[0 0 1 1-e 0+e 0+e],c2);patch([0 0 1 1-e 0+e 0+e],[0 1 1 1-e 1-e 0+e],c3);plot([0 1 1 0 0],[0 0 1 1 0]);
  wires:
  "p{2}"/1 -> mux/1
  mux/1 -> "pd{2,1}"/1
